simulink model "IMU_Filter_Model"  (R2019a)
settings: Solver=VariableStepAuto  StartTime=0.0  StopTime=10.0  RelTol=1e-3
settings Model: Creator=ABHI  LastModifiedBy=ABHI

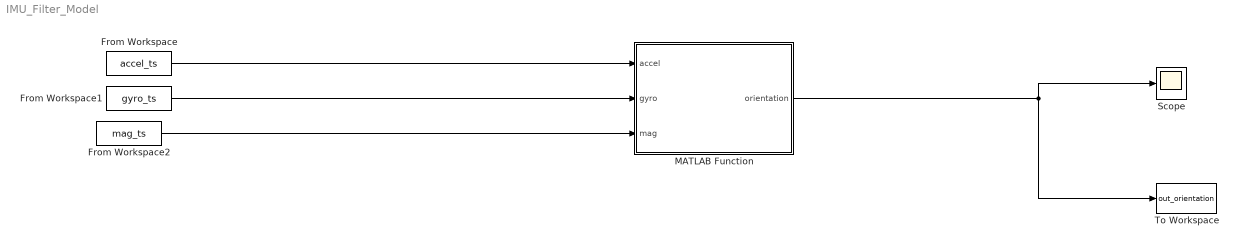
== system IMU_Filter_Model ==
  From Workspace : FromWorkspace  VariableName=accel_ts  SampleTime=0
  From Workspace1 : FromWorkspace  VariableName=gyro_ts  SampleTime=0
  From Workspace2 : FromWorkspace  VariableName=mag_ts  SampleTime=0
  MATLAB Function : MATLAB Function  TreatAsAtomicUnit=on
  Scope : Scope
  To Workspace : ToWorkspace  VariableName=out_orientation  SaveFormat=Timeseries  SampleTime=-1
  wires:
  MATLAB Function/1(orientation) -> To Workspace/1, Scope/1
  From Workspace/1 -> MATLAB Function/1(accel)
  From Workspace2/1 -> MATLAB Function/3(mag)
  From Workspace1/1 -> MATLAB Function/2(gyro)

== matlab function IMU_Filter_Model/MATLAB Function ==
  data: accel input; orientation output; gyro input; mag input
function orientation = fusion_filter(accel, gyro, mag)
    % Pre-allocate output size for Simulink compiler
    orientation = zeros(3, 1);

    dt = 0.01;      % Time step (seconds)
    alpha = 0.98;   % Filter weighting factor (0.98 gyro, 0.02 accel/mag)

    persistent roll pitch yaw
    if isempty(roll)
        roll = 0; 
        pitch = 0; 
        yaw = 0;
    end

    % 1. Calculate Roll & Pitch from Accelerometer (degrees)
    ax = accel(1); ay = accel(2); az = accel(3);
    roll_acc  = atan2(ay, az) * (180/pi);
    pitch_acc = atan2(-ax, sqrt(ay^2 + az^2)) * (180/pi);

    % 2. Convert Gyro Angular Rates to degrees/sec
    gx = gyro(1) * (180/pi);
    gy = gyro(2) * (180/pi);
    gz = gyro(3) * (180/pi);

    % 3. Calculate Heading (Yaw reference) from Magnetometer (degrees)
    mx = mag(1); my = mag(2);
    yaw_mag = atan2(-my, mx) * (180/pi);

    % 4. 9-DOF Complementary Filter Fusion
    roll  = alpha * (roll + gx * dt)  + (1 - alpha) * roll_acc;
    pitch = alpha * (pitch + gy * dt) + (1 - alpha) * pitch_acc;
    yaw   = alpha * (yaw + gz * dt)   + (1 - alpha) * yaw_mag;

    % Output vector [Roll; Pitch; Yaw]
    orientation = [roll; pitch; yaw];
end
